simulink model "LQR_EX"  (Simulink 6.6)
settings: Solver=ode45  StartTime=0.0  StopTime=2  MaxStep=1e-3  RelTol=1e-3
values from neighbouring files (symbols this model uses):
  K1 = K(1,1)    [file_for_LQR_EX.m]
  K2 = K(1,2)    [file_for_LQR_EX.m]
libraries: simulink x1
settings Model: Creator=Thomas Chmielewski  LastModifiedBy=Thomas Chmielewski
settings DataIOCC: SignalLoggingName=sigsOut
settings DebuggingCC: SignalResolutionControl=TryResolveAllWithWarning  SolverPrmCheckMsg=none  MultiTaskDSMMsg=warning  MultiTaskCondExecSysMsg=none  StrictBusMsg=None
settings HardwareCC: TargetUnknown=on
settings RTWCC: IncludeERTFirstTime=on
settings GRTTargetCC: ModelReferenceCompliant=off  MatFileLogging=off

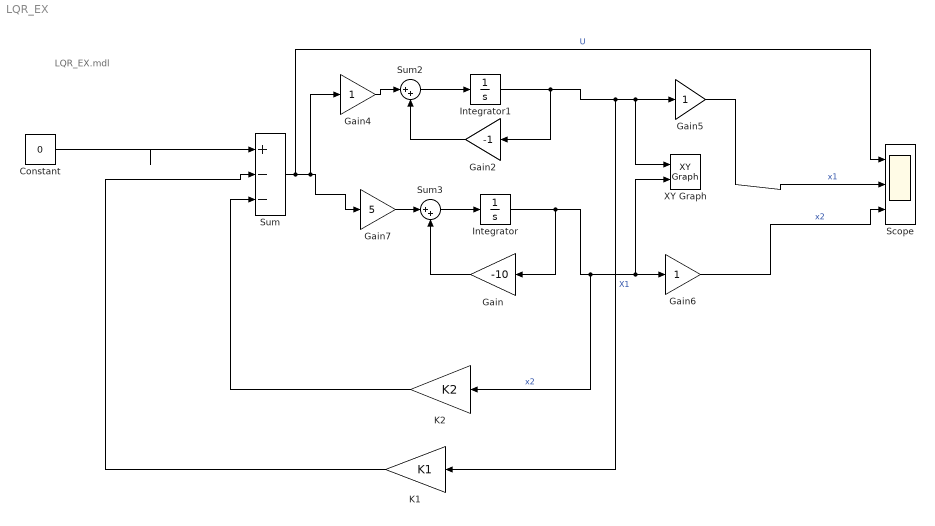
== system LQR_EX ==
  note: LQR_EX.mdl
  Constant : Constant  Value=0
  Gain : Gain  Orientation=left  Gain=-10  SaturateOnIntegerOverflow=on
  Gain2 : Gain  Orientation=left  Gain=-1  SaturateOnIntegerOverflow=on
  Gain4 : Gain  SaturateOnIntegerOverflow=on
  Gain5 : Gain  SaturateOnIntegerOverflow=on
  Gain6 : Gain  SaturateOnIntegerOverflow=on
  Gain7 : Gain  Gain=5  SaturateOnIntegerOverflow=on
  Integrator : Integrator  InitialCondition=10
  Integrator1 : Integrator  InitialCondition=10
  K1 : Gain  Orientation=left  Gain=K1  SaturateOnIntegerOverflow=on
  K2 : Gain  Orientation=left  Gain=K2  SaturateOnIntegerOverflow=on
  Scope : Scope  NumInputPorts=3
      settings: YMin=-4.5e-071~1.25673e-088~-6e-069  YMax=4.02153e-087~5e-072~5.14756e-085
  Sum : Sum  Inputs=|+--  SaturateOnIntegerOverflow=on
  Sum2 : Sum  Inputs=|++  SaturateOnIntegerOverflow=on
  Sum3 : Sum  Inputs=|++  SaturateOnIntegerOverflow=on
  XY Graph : simulink/Sinks/XY Graph  SystemSampleTime=-1  xmin=-10  xmax=10  ymin=-10  ymax=10  st=-1
  wires:
  Gain5/1 -> Scope/2  "x1"
  Gain6/1 -> Scope/3  "x2"
  Integrator1/1 -> Gain2/1, K1/1, Gain5/1, XY Graph/1  "X1"
  Integrator/1 -> Gain/1, K2/1, Gain6/1, XY Graph/2  "x2"
  Sum/1 -> Gain7/1, Gain4/1, Scope/1  "U"
  K1/1 -> Sum/2
  Sum3/1 -> Integrator/1
  Gain/1 -> Sum3/2
  Sum2/1 -> Integrator1/1
  Gain2/1 -> Sum2/2
  Gain7/1 -> Sum3/1
  Gain4/1 -> Sum2/1
  K2/1 -> Sum/3
  Constant/1 -> Sum/1
